simulink model "week1_2"  (R2020b)
settings: Solver=VariableStepAuto  StartTime=0.0  StopTime=100  RelTol=1e-3
PreLoadFcn:
  | clc;
  | close all;
  | clear all;
  | m1=465;
  | m2=135;
  | k1=5700;
  | k2=135;
  | b=290;
  | F=1;
settings Model: Creator=hp  LastModifiedBy=ASUS

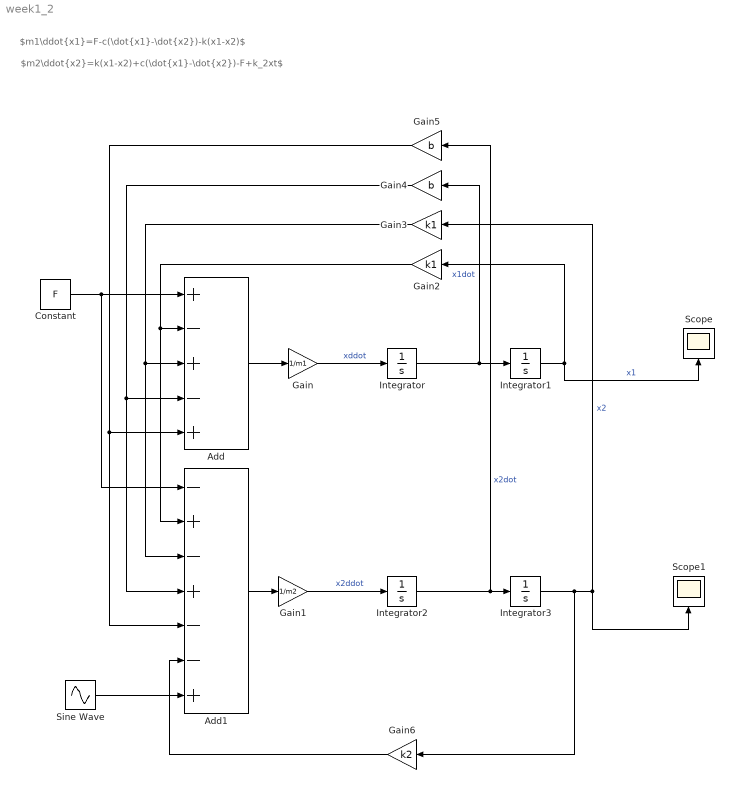
== system week1_2 ==
  note: $m2\ddot{x2}=k(x1-x2)+c(\dot{x1}-\dot{x2})-F+k_2xt$
  note: $m1\ddot{x1}=F-c(\dot{x1}-\dot{x2})-k(x1-x2)$
  Add : Sum  Inputs=+-+-+
  Add1 : Sum  Inputs=-+-+--+
  Constant : Constant  Value=F
  Gain : Gain  Gain=1/m1
  Gain1 : Gain  Gain=1/m2
  Gain2 : Gain  Gain=k1
  Gain3 : Gain  Gain=k1
  Gain4 : Gain  Gain=b
  Gain5 : Gain  Gain=b
  Gain6 : Gain  Gain=k2
  Integrator{,1..3} (4 alike) : Integrator
  Scope : Scope
  Scope1 : Scope
  Sine Wave : Sin  SampleTime=0
  wires:
  Gain4/1 -> Add1/4, Add/4
  Gain3/1 -> Add1/3, Add/3
  Integrator1/1 -> Scope/1, Gain2/1  "x1"
  Add/1 -> Gain/1
  Integrator/1 -> Gain4/1, Integrator1/1  "x1dot"
  Integrator3/1 -> Gain6/1, Gain3/1, Scope1/1  "x2"
  Gain1/1 -> Integrator2/1  "x2ddot"
  Integrator2/1 -> Gain5/1, Integrator3/1  "x2dot"
  Gain/1 -> Integrator/1  "xddot"
  Gain2/1 -> Add1/2, Add/2
  Constant/1 -> Add1/1, Add/1
  Gain6/1 -> Add1/6
  Gain5/1 -> Add1/5, Add/5
  Add1/1 -> Gain1/1
  Sine Wave/1 -> Add1/7
